simulink model "basic_acc"  (R2022a)
settings: Solver=VariableStepAuto  StartTime=0.0  StopTime=50  RelTol=1e-3
libraries: vrlib x2, simulink x1, mpcadaslib x1
settings Model: Creator=jjworklab  LastModifiedBy=jjworklab

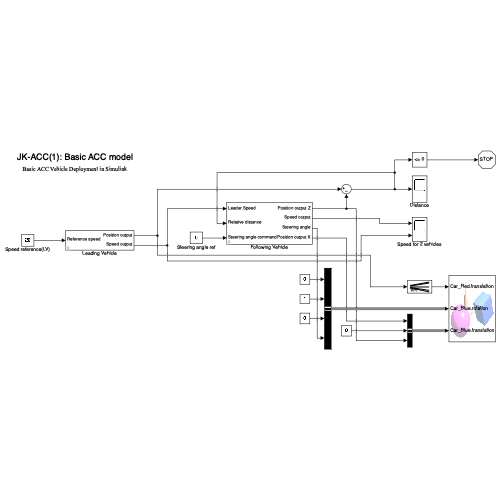
[thumbnail: Simulink's stored preview of the top-level diagram]
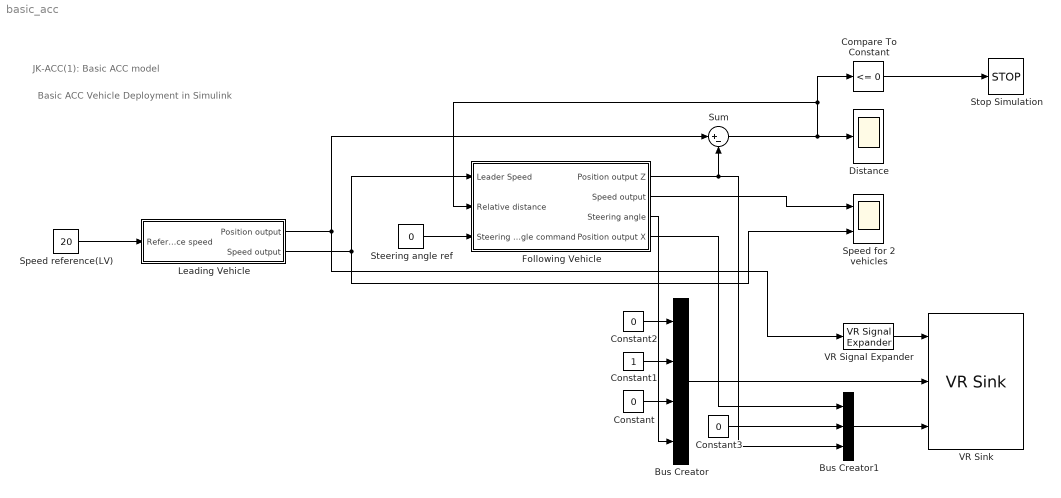
== system basic_acc ==
  note: Basic ACC Vehicle Deployment in Simulink
  note: JK-ACC(1): Basic ACC model
  Bus Creator : BusCreator  Inputs=4
  Bus Creator1 : BusCreator  Inputs=3
  Compare To Constant : simulink/Logic and Bit Operations/Compare To Constant  relop=<=  const=0  OutDataTypeStr=boolean
  Constant : Constant  Value=0
  Constant1 : Constant
  Constant2 : Constant  Value=0
  Constant3 : Constant  Value=0
  Distance : Scope
  Following Vehicle : Subsystem  mask{Value1=0, Value2=30}
      mask prompts: Value1 "Initial position"; Value2 "Initial speed"
      mask TypeOptions Value1: Initial position Z/Value
      mask TypeOptions Value2: Initial speed/Value
  Leading Vehicle : Subsystem  mask{Value1=25, Value2=20}
      mask prompts: Value1 "Initial position"; Value2 "Initial speed"
      mask TypeOptions Value1: Initial position/Value
      mask TypeOptions Value2: Initial speed/Value
  Speed for 2 vehicles : Scope  NumInputPorts=2
  Speed reference(LV) : Constant  Value=20
  Steering angle ref : Constant  Value=0
  Stop Simulation : Stop
  Sum : Sum  Inputs=|+-
  VR Signal Expander : vrlib/VR Signal Expander  outwidth=3  outidx=[3]
  VR Sink : vrlib/VR Sink  InstantiateOnLoad=on  SampleTime=0.1  ViewEnable=on  RemoteChange=off  RemoteView=off  FieldsWritten=Car_Red.translation.3.1.1.double#Car_Blue.rotation.4.1.1.double#Car_Blue.translation.3.1.1.double  WorldFileName=PlatoonWorld.WRL  AutoView=off  VideoDimensions=[]  AllowVariableSize=off
  wires:
  Speed reference(LV)/1 -> Leading Vehicle/1(Reference speed)
  Following Vehicle/1(Position output Z) -> Bus Creator1/3, Sum/2
  Leading Vehicle/1(Position output) -> VR Signal Expander/1, Sum/1
  Following Vehicle/2(Speed output) -> Speed for 2 vehicles/1
  Leading Vehicle/2(Speed output) -> Following Vehicle/1(Leader Speed), Speed for 2 vehicles/2
  Sum/1 -> Distance/1, Following Vehicle/2(Relative distance), Compare To Constant/1
  Compare To Constant/1 -> Stop Simulation/1
  Steering angle ref/1 -> Following Vehicle/3(Steering angle command)
  VR Signal Expander/1 -> VR Sink/1
  Following Vehicle/3(Steering angle) -> Bus Creator/4
  Constant/1 -> Bus Creator/3
  Constant1/1 -> Bus Creator/2
  Constant2/1 -> Bus Creator/1
  Bus Creator/1 -> VR Sink/2
  Following Vehicle/4(Position output X) -> Bus Creator1/1
  Constant3/1 -> Bus Creator1/2
  Bus Creator1/1 -> VR Sink/3

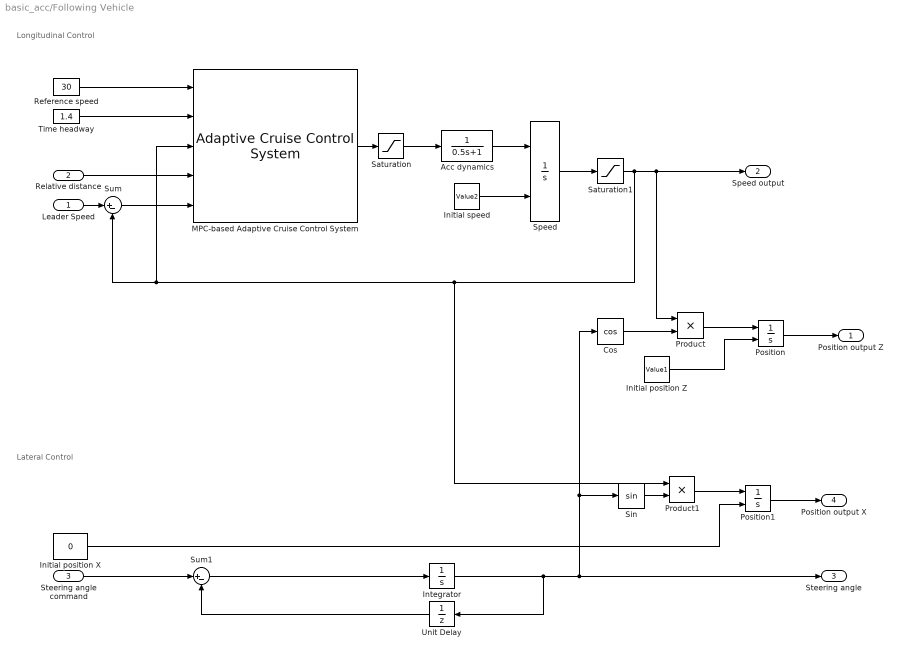
== system basic_acc/Following Vehicle ==
  note: Longitudinal Control
  note: Lateral Control
  Leader Speed : Inport
  Relative distance : Inport  Port=2
  Steering angle command : Inport  Port=3
  Acc dynamics : TransferFcn  Denominator=[0.5 1]
  Cos : Trigonometry  Operator=cos
  Initial position X : Constant  Value=0
  Initial position Z : Constant  Value=Value1
  Initial speed : Constant  Value=Value2
  Integrator : Integrator
  MPC-based Adaptive Cruise Control System : mpcadaslib/Adaptive Cruise Control System  EgoModel=tf(1,[0.5,1,0])  InitialEgoVelocity=30  DefaultSpacing=10  MaxVelocity=50  MinAcceleration=-3  amin_ext=off  MaxAcceleration=2  amax_ext=off  Ts=0.5  PredictionHorizon=200  ControllerBehavior=0.6  suboptimal=off  maxiter=10  datatypeopt=double  optmode=off  trackmode=off
  Position : Integrator  InitialConditionSource=external
  Position1 : Integrator  InitialConditionSource=external
  Product : Product
  Product1 : Product
  Reference speed : Constant  Value=30
  Saturation : Saturate  UpperLimit=2  LowerLimit=-3
  Saturation1 : Saturate  UpperLimit=inf  LowerLimit=0
  Sin : Trigonometry
  Speed : Integrator  InitialConditionSource=external
  Sum : Sum  Inputs=|+-
  Sum1 : Sum  Inputs=|+-
  Time headway : Constant  Value=1.4
  Unit Delay : UnitDelay  SampleTime=-1  HasFrameUpgradeWarning=on
  Position output Z : Outport
  Speed output : Outport  Port=2
  Steering angle : Outport  Port=3
  Position output X : Outport  Port=4
  wires:
  Position/1 -> Position output Z/1
  Initial position Z/1 -> Position/2
  Saturation/1 -> Acc dynamics/1
  Saturation1/1 -> Product1/1, MPC-based Adaptive Cruise Control System/3, Sum/2, Speed output/1, Product/1
  Acc dynamics/1 -> Speed/1
  Initial speed/1 -> Speed/2
  Speed/1 -> Saturation1/1
  Sum/1 -> MPC-based Adaptive Cruise Control System/5
  Leader Speed/1 -> Sum/1
  Relative distance/1 -> MPC-based Adaptive Cruise Control System/4
  Time headway/1 -> MPC-based Adaptive Cruise Control System/2
  Reference speed/1 -> MPC-based Adaptive Cruise Control System/1
  MPC-based Adaptive Cruise Control System/1 -> Saturation/1
  Steering angle command/1 -> Sum1/1
  Integrator/1 -> Unit Delay/1, Steering angle/1, Sin/1, Cos/1
  Sum1/1 -> Integrator/1
  Unit Delay/1 -> Sum1/2
  Initial position X/1 -> Position1/2
  Cos/1 -> Product/2
  Product/1 -> Position/1
  Sin/1 -> Product1/2
  Product1/1 -> Position1/1
  Position1/1 -> Position output X/1

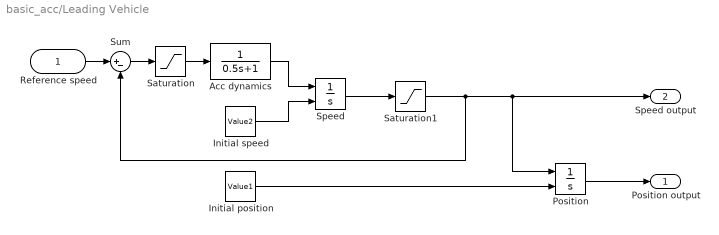
== system basic_acc/Leading Vehicle ==
  Reference speed : Inport
  Acc dynamics : TransferFcn  Denominator=[0.5 1]
  Initial position : Constant  Value=Value1
  Initial speed : Constant  Value=Value2
  Position : Integrator  InitialConditionSource=external
  Saturation : Saturate  UpperLimit=2  LowerLimit=-3
  Saturation1 : Saturate  UpperLimit=inf  LowerLimit=0
  Speed : Integrator  InitialConditionSource=external
  Sum : Sum  Inputs=|+-
  Position output : Outport
  Speed output : Outport  Port=2
  wires:
  Position/1 -> Position output/1
  Initial position/1 -> Position/2
  Saturation/1 -> Acc dynamics/1
  Saturation1/1 -> Speed output/1, Position/1, Sum/2
  Acc dynamics/1 -> Speed/1
  Initial speed/1 -> Speed/2
  Speed/1 -> Saturation1/1
  Sum/1 -> Saturation/1
  Reference speed/1 -> Sum/1
